simulink model "dofAutopilot2"  (R2024b)
settings: Solver=ode4  StartTime=0.0  StopTime=30  FixedStep=0.01  RelTol=1e-3
undefined symbols (not defined in the file or in its folder): D, L, T, W
libraries: shared6dof x1, slpidlib x1
settings Model: Creator=sahil  LastModifiedBy=sahil

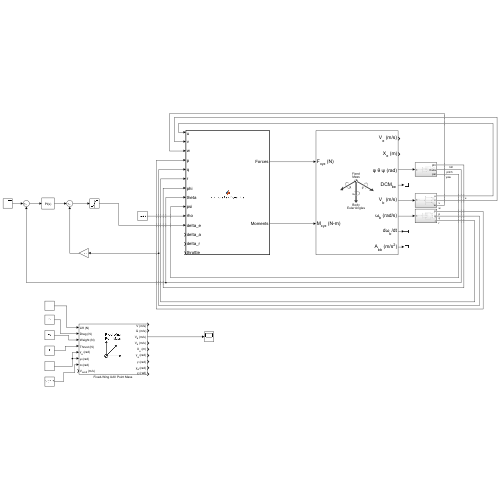
[thumbnail: Simulink's stored preview of the top-level diagram]
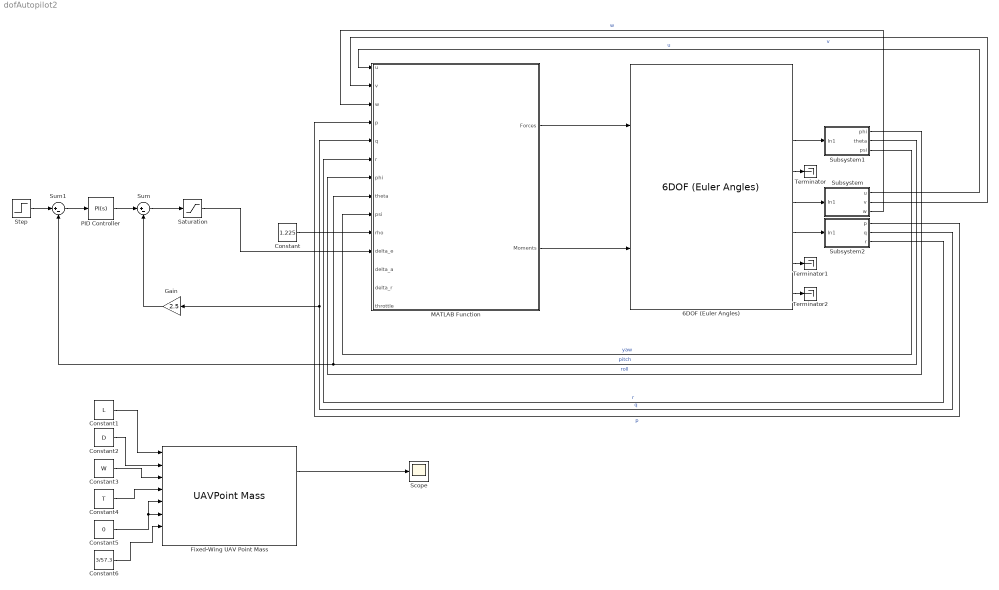
== system dofAutopilot2 ==
  6DOF (Euler Angles) : shared6dof/6DOF (Euler Angles)  units=Metric (MKS)  mtype=Fixed  rep=Euler Angles  xme_0=[0 0 -100]  Vm_0=[15 0 0]  eul_0=[0 0.05 0]  pm_0=[0 0 0]  mass_0=13.5  mass_e=0.5  mass_f=2.0  inertia=[0.824,0, 0.120;0,1.135,0;0.120, 0,1.759]  inertia_e=eye(3)  inertia_f=2*eye(3)  k_quat=1.0  vre_flag=on  abi_flag=off  aMode=0  xme_statename=''  Vm_statename=''  eul_statename=''  quat_statename=''  pm_statename=''  mass_statename=''
  Constant : Constant  Value=1.225
  Constant1 : Constant  Value=L
  Constant2 : Constant  Value=D
  Constant3 : Constant  Value=W
  Constant4 : Constant  Value=T
  Constant5 : Constant  Value=0
  Constant6 : Constant  Value=3/57.3
  Fixed-Wing UAV Point Mass : UAVPointMass  altitude=100  airspeed=V
  Gain : Gain  Gain=2.5
  MATLAB Function : MATLAB Function  TreatAsAtomicUnit=on
  PID Controller : slpidlib/PID Controller  Controller=PI  Form=Parallel  TimeDomain=Continuous-time  UseExternalTs=off  SampleTime=-1  IntegratorMethod=Forward Euler  FilterMethod=Forward Euler  ControllerParametersSource=internal  P=0.1  I=0  UseKiTs=off  D=-19.1481496981679  UseExternalDerivativeSource=off  N=8783.15164957376  UseFilter=on  TunerSelectOption=Transfer Function Based (PID Tuner App)  InitialConditionSource=internal  InitialConditionForIntegrator=0  InitialConditionForFilter=0  DifferentiatorICPrevScaledInput=0  ExternalReset=none  TrackingMode=off  Kt=1  LimitOutput=off  SatLimitsSource=internal  UpperSaturationLimit=inf  LowerSaturationLimit=-inf  LinearizeAsGain=on  AntiWindupMode=none  Kb=1  LimitIntegrator=off  UpperIntegratorSaturationLimit=inf  LowerIntegratorSaturationLimit=-inf  POutMin=[]  POutMax=[]  IOutMin=[]  IOutMax=[]  DOutMin=[]  DOutMax=[]  NOutMin=[]  NOutMax=[]  SumOutMin=[]  SumOutMax=[]  SaturationOutMin=[]  SaturationOutMax=[]  PParamMin=[]  PParamMax=[]  IParamMin=[]  IParamMax=[]  DParamMin=[]  DParamMax=[]  NParamMin=[]  NParamMax=[]  KbParamMin=[]  KbParamMax=[]  KtParamMin=[]  KtParamMax=[]  KbOutMin=[]  KbOutMax=[]  KtOutMin=[]  KtOutMax=[]  IntegratorOutMin=[]  IntegratorOutMax=[]  FilterOutMin=[]  FilterOutMax=[]  SumI1OutMin=[]  SumI1OutMax=[]  SumI2OutMin=[]  SumI2OutMax=[]  SumI3OutMin=[]  SumI3OutMax=[]  SumI4OutMin=[]  SumI4OutMax=[]  SumDOutMin=[]  SumDOutMax=[]  DifferentiatorOutMin=[]  DifferentiatorOutMax=[]  FilterDiffOutCoefMin=[]  FilterDiffOutCoefMax=[]  ReciprocalOutMin=[]  ReciprocalOutMax=[]  SumDenOutMin=[]  SumDenOutMax=[]  SumNumOutMin=[]  SumNumOutMax=[]  DivideOutMin=[]  DivideOutMax=[]  UdiffTsProdOutMin=[]  UdiffTsProdOutMax=[]  NTsProdOutMin=[]  NTsProdOutMax=[]  UintegralTsProdOutMin=[]  UintegralTsProdOutMax=[]  UngainTsProdOutMin=[]  UngainTsProdOutMax=[]  ClampingZeroOutDataTypeStr=Inherit: Inherit via back propagation  ClampingZeroOutMin=[]  ClampingZeroOutMax=[]  FilterDenConstantOutDataTypeStr=Inherit: Inherit via back propagation  FilterDenConstantOutMin=[]  FilterDenConstantOutMax=[]  PCopyOutDataTypeStr=Inherit: Inherit via back propagation  PCopyOutMin=[]  PCopyOutMax=[]  NCopyOutDataTypeStr=Inherit: Inherit via back propagation  NCopyOutMin=[]  NCopyOutMax=[]  IntegratorContinuousStateAttributes=''  IntegratorStateMustResolveToSignalObject=off  IntegratorRTWStateStorageClass=Auto  FilterContinuousStateAttributes=''  FilterStateMustResolveToSignalObject=off  FilterRTWStateStorageClass=Auto  ParallelPVariant=InternalParameters  IdealPVariant=Disabled  IVariant=InternalParameters  DVariant=Disabled  IntegratorVariant=Continuous  SatVariant=Disabled  AWVariant=Passthrough  PCopyVariant=Disabled  TRVariant=Disabled  FdbkBlocksVariant=Forward  IdealPFdbkVariant=Disabled  SatFdbkVariant=Disabled  DerivativeFilterVariant=Disabled  NVariant=Disabled  NCopyVariant=Disabled_SignalSpec  FilterICVariant=Disabled  IntegratorICVariant=InternalICs  ExternalResetVariant=Disabled  TRSumVariant=Passthrough  SumFdbkVariant=Disabled  SumVariant=Sum_PI  TsampFilterVariant=InternalTs  TsampNgainVariant=Passthrough  TsampIntegralVariant=Disabled_SignalSpec  ExternalSaturationOutDataTypeStr=Inherit: Same as second input  DerivativeSourceVariant=Disabled  PreIntVariant=InternalPreInt
  Saturation : Saturate  UpperLimit=25/57.3  LowerLimit=-25/57.3
  Scope : Scope
  Step : Step  After=5/57.3  SampleTime=0
  Subsystem : Subsystem
  Subsystem1 : Subsystem
  Subsystem2 : Subsystem
  Sum : Sum  Inputs=|+-
  Sum1 : Sum  Inputs=|+-
  Terminator : Terminator
  Terminator1 : Terminator
  Terminator2 : Terminator
  wires:
  Constant/1 -> MATLAB Function/10(rho)
  MATLAB Function/1(Forces) -> 6DOF (Euler Angles)/1
  MATLAB Function/2(Moments) -> 6DOF (Euler Angles)/2
  6DOF (Euler Angles)/5 -> Subsystem/1(In1)
  6DOF (Euler Angles)/3 -> Subsystem1/1(In1)
  6DOF (Euler Angles)/6 -> Subsystem2/1(In1)
  6DOF (Euler Angles)/4 -> Terminator/1
  6DOF (Euler Angles)/7 -> Terminator1/1
  6DOF (Euler Angles)/8 -> Terminator2/1
  Subsystem/1(u) -> MATLAB Function/1(u)  "u"
  Subsystem/2(v) -> MATLAB Function/2(v)  "v"
  Subsystem/3(w) -> MATLAB Function/3(w)  "w"
  Subsystem2/1(p) -> MATLAB Function/4(p)  "p"
  Subsystem2/2(q) -> Gain/1, MATLAB Function/5(q)  "q"
  Subsystem2/3(r) -> MATLAB Function/6(r)  "r"
  Subsystem1/1(phi) -> MATLAB Function/7(phi)  "roll"
  Subsystem1/2(theta) -> Sum1/2, MATLAB Function/8(theta)  "pitch"
  Subsystem1/3(psi) -> MATLAB Function/9(psi)  "yaw"
  Sum/1 -> Saturation/1
  Step/1 -> Sum1/1
  Sum1/1 -> PID Controller/1
  PID Controller/1 -> Sum/1
  Gain/1 -> Sum/2
  Saturation/1 -> MATLAB Function/11(delta_e)
  Constant1/1 -> Fixed-Wing UAV Point Mass/1
  Constant2/1 -> Fixed-Wing UAV Point Mass/2
  Constant3/1 -> Fixed-Wing UAV Point Mass/3
  Constant4/1 -> Fixed-Wing UAV Point Mass/4
  Constant5/1 -> Fixed-Wing UAV Point Mass/6, Fixed-Wing UAV Point Mass/5
  Constant6/1 -> Fixed-Wing UAV Point Mass/7
  Fixed-Wing UAV Point Mass/3 -> Scope/1

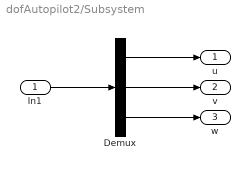
== system dofAutopilot2/Subsystem ==
  In1 : Inport
  Demux : Demux  Outputs=3
  u : Outport
  v : Outport  Port=2
  w : Outport  Port=3
  wires:
  In1/1 -> Demux/1
  Demux/3 -> w/1
  Demux/1 -> u/1
  Demux/2 -> v/1

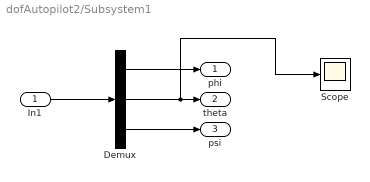
== system dofAutopilot2/Subsystem1 ==
  In1 : Inport
  Demux : Demux  Outputs=3
  Scope : Scope
  phi : Outport
  theta : Outport  Port=2
  psi : Outport  Port=3
  wires:
  Demux/2 -> Scope/1, theta/1
  Demux/1 -> phi/1
  Demux/3 -> psi/1
  In1/1 -> Demux/1

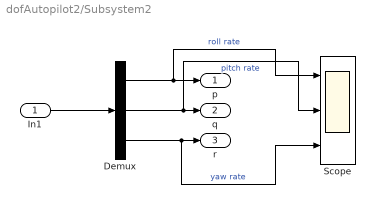
== system dofAutopilot2/Subsystem2 ==
  In1 : Inport
  Demux : Demux  Outputs=3
  Scope : Scope  NumInputPorts=3
  p : Outport
  q : Outport  Port=2
  r : Outport  Port=3
  wires:
  In1/1 -> Demux/1
  Demux/3 -> Scope/3, r/1  "yaw rate"
  Demux/1 -> Scope/1, p/1  "roll rate"
  Demux/2 -> Scope/2, q/1  "pitch rate"

== matlab function dofAutopilot2/MATLAB Function ==
  data: u input; Forces output; v input; w input; p input; q input; r input; phi input; theta input; psi input; rho input; delta_e input; delta_a input; delta_r input; throttle input; Moments output
function [Forces, Moments] = computeAeroDynamics( ...
    u, v, w, p, q, r, ...
    phi, theta, psi, ...
    rho, delta_e, delta_a, delta_r, throttle)

%% =============================
% 1. Aircraft Parameters
%% =============================
m = 13.5;      % kg
g = 9.81;      % m/s^2

S = 0.55;      % m^2
b = 2.895;     % m
c = 0.1899;    % m

%% =============================
% 2. Air Data
%% =============================
V = sqrt(u^2 + v^2 + w^2);
V = max(V, 0.1);   % avoid division by zero

alpha = atan2(w, u);
beta  = asin(max(min(v / V, 1), -1));

q_bar = 0.5 * rho * V^2;

% Allow wider alpha range for stability
alpha = max(min(alpha, deg2rad(25)), -deg2rad(25));

%% =============================
% 3. Aerodynamic Coefficients
%% =============================

% ---- Longitudinal ----
CL0  = 0.28;
CLa  = 5.5;
CLq  = 6.0;
CLde = 0.3;

CD0 = 0.03;
K   = 0.06;

Cm0  = 0.0;
Cma  = -2.5;
Cmq  = -20;
Cmde = -1.2;   % ✔ consistent sign: +δe → nose DOWN

% ---- Lateral-directional ----
CYb  = -0.2;
CYdr = 0.2;

Clb  = -0.12;
Clp  = -0.5;
Clr  = 0.25;
Clda = 0.08;

Cnb  = 0.06;
Cnr  = -0.1;
Cndr = -0.05;

%% =============================
% 4. Non-dimensional Coefficients
%% =============================

q_hat = q*c/(2*V);
p_hat = p*b/(2*V);
r_hat = r*b/(2*V);

% Clamp rates to avoid blow-up
q_hat = max(min(q_hat, 5), -5);
p_hat = max(min(p_hat, 5), -5);
r_hat = max(min(r_hat, 5), -5);

CL = CL0 + CLa*alpha + CLq*q_hat + CLde*delta_e;
CD = CD0 + K*(CL^2);
Cm = Cm0 + Cma*alpha + Cmq*q_hat + Cmde*delta_e;

CY = CYb*beta + CYdr*delta_r;

Cl = Clb*beta + Clp*p_hat + Clr*r_hat + Clda*delta_a;
Cn = Cnb*beta + Cnr*r_hat + Cndr*delta_r;

%% =============================
% 5. Aerodynamic Forces (Body Axes)
%% =============================

L = q_bar * S * CL;
D = q_bar * S * CD;
Y = q_bar * S * CY;

% Wind → Body (Z-down convention)
Fx_aero = -D*cos(alpha)*cos(beta) ...
          + Y*sin(beta) ...
          + L*sin(alpha)*cos(beta);

Fy_aero = -D*cos(alpha)*sin(beta) ...
          + Y*cos(beta) ...
          + L*sin(alpha)*sin(beta);

Fz_aero = -L*cos(alpha) - D*sin(alpha);  % ✔ Lift acts upward (−Z)

%% =============================
% 6. Moments
%% =============================

Mx = q_bar * S * b * Cl;
My = q_bar * S * c * Cm;
Mz = q_bar * S * b * Cn;

%% =============================
% 7. Propulsion
%% =============================

max_thrust = 80;

% Keep thrust always available (important)
Thrust = max_thrust * throttle * (0.3 + 0.7*(1 - V/30));
Thrust = max(0, Thrust);

Fx_prop = Thrust;
Fy_prop = 0;
Fz_prop = 0;

% Small thrust offset (optional)
r_thrust = [0; 0; 0.05];
M_prop = cross(r_thrust, [Fx_prop; Fy_prop; Fz_prop]);

%% =============================
% 8. Gravity (Body Frame, Z-down)
%% =============================

Fg = m * g * [
    -sin(theta);
     sin(phi)*cos(theta);
     cos(phi)*cos(theta)
];

%% =============================
% 9. Total Forces & Moments
%% =============================

Fx = Fx_aero + Fx_prop + Fg(1);
Fy = Fy_aero + Fy_prop + Fg(2);
Fz = Fz_aero + Fz_prop + Fg(3);

Mx = Mx + M_prop(1);
My = My + M_prop(2);
Mz = Mz + M_prop(3);

Forces  = [Fx; Fy; Fz];
Moments = [Mx; My; Mz];

end
